simulink model "Complete_Sensorless_FOC_EKF_simulink_model"  (R2026a)
settings: Solver=ode23s  StopTime=inf  FixedStep=5e-5  MaxStep=1e-2
model workspace (MAT data in the model file):
  SL_ROS_VariableLengthArrays_MaxSizes : object (value not decoded)
values from neighbouring files (symbols this model uses):
  id_ref = 0    [motor_params.m]
  J = 0.001    [motor_params.m]
  Kp_id = 37.7    [motor_params.m]
  Kp_iq = 65.97    [motor_params.m]
  lam = 0.175    [motor_params.m]
  Ld = 6e-3    (= 0.006)    [motor_params.m]
  Lq = 10.5e-3    (= 0.0105)    [motor_params.m]
  Ts = 50e-6    (= 5e-05)    [motor_params.m]
  V_dc = 48    [motor_params.m]
  V_lim = 27.7    [motor_params.m]
undefined symbols (not defined in the file or in its folder): data, data_SL_Info, DiscIntNeverNeededParam, dspblkCoreblockFVToolHelper, gcbh
libraries: nesl_utility x34, fl_lib x22, ee_lib x16, ros2lib x3
(part 2 of 2)

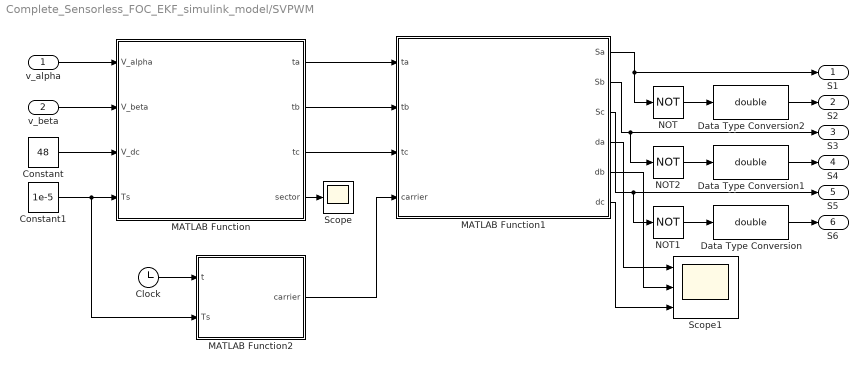
== system Complete_Sensorless_FOC_EKF_simulink_model/SVPWM ==
  v_alpha : Inport
  v_beta : Inport  Port=2
  Clock : Clock
  Constant : Constant  Value=48
  Constant1 : Constant  Value=1e-5
  Data Type Conversion : DataTypeConversion  OutDataTypeStr=double  SaturateOnIntegerOverflow=off  RndMeth=Floor
  Data Type Conversion1 : DataTypeConversion  OutDataTypeStr=double  SaturateOnIntegerOverflow=off  RndMeth=Floor
  Data Type Conversion2 : DataTypeConversion  OutDataTypeStr=double  SaturateOnIntegerOverflow=off  RndMeth=Floor
  MATLAB Function : MATLAB Function  TreatAsAtomicUnit=on
  MATLAB Function1 : MATLAB Function  TreatAsAtomicUnit=on
  MATLAB Function2 : MATLAB Function  TreatAsAtomicUnit=on
  NOT : Logic  Operator=NOT  IconShape=distinctive  AllPortsSameDT=off  OutDataTypeStr=boolean
  NOT1 : Logic  Operator=NOT  IconShape=distinctive  AllPortsSameDT=off  OutDataTypeStr=boolean
  NOT2 : Logic  Operator=NOT  IconShape=distinctive  AllPortsSameDT=off  OutDataTypeStr=boolean
  Scope : Scope
      settings: ActiveDisplayYMinimum=-1.4009794226019459  ActiveDisplayYMaximum=12.404458534659673
  Scope1 : Scope  NumInputPorts=3
      settings: ActiveDisplayYMinimum=-0.1185846672948957  ActiveDisplayYMaximum=0.92580647336062072  DataLoggingVariableName=ScopeData9
  S1 : Outport
  S2 : Outport  Port=2
  S3 : Outport  Port=3
  S4 : Outport  Port=4
  S5 : Outport  Port=5
  S6 : Outport  Port=6
  wires:
  v_alpha/1 -> MATLAB Function/1(V_alpha)
  v_beta/1 -> MATLAB Function/2(V_beta)
  Constant/1 -> MATLAB Function/3(V_dc)
  Constant1/1 -> MATLAB Function2/2(Ts), MATLAB Function/4(Ts)
  Clock/1 -> MATLAB Function2/1(t)
  MATLAB Function/1(ta) -> MATLAB Function1/1(ta)
  MATLAB Function/2(tb) -> MATLAB Function1/2(tb)
  MATLAB Function/3(tc) -> MATLAB Function1/3(tc)
  MATLAB Function2/1(carrier) -> MATLAB Function1/4(carrier)
  MATLAB Function1/2(Sb) -> NOT2/1, S3/1
  NOT/1 -> Data Type Conversion2/1
  NOT2/1 -> Data Type Conversion1/1
  NOT1/1 -> Data Type Conversion/1
  MATLAB Function/4(sector) -> Scope/1
  Data Type Conversion2/1 -> S2/1
  Data Type Conversion1/1 -> S4/1
  Data Type Conversion/1 -> S6/1
  MATLAB Function1/1(Sa) -> NOT/1, S1/1
  MATLAB Function1/3(Sc) -> NOT1/1, S5/1
  MATLAB Function1/4(da) -> Scope1/1
  MATLAB Function1/5(db) -> Scope1/2
  MATLAB Function1/6(dc) -> Scope1/3

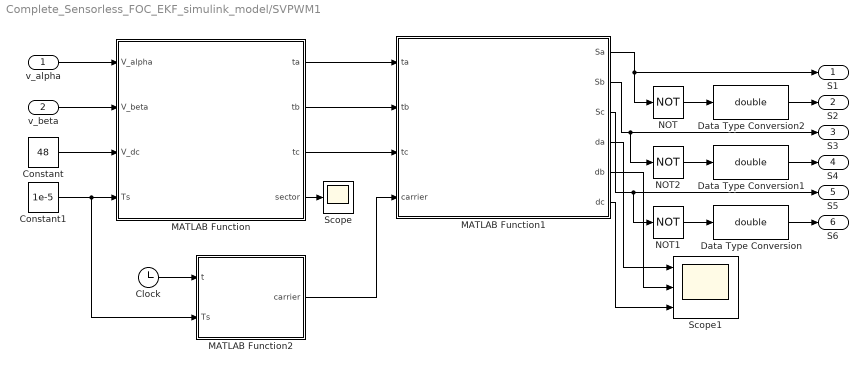
== system Complete_Sensorless_FOC_EKF_simulink_model/SVPWM1 ==
  v_alpha : Inport
  v_beta : Inport  Port=2
  Clock : Clock
  Constant : Constant  Value=48  SampleTime=-1
  Constant1 : Constant  Value=1e-5
  Data Type Conversion : DataTypeConversion  OutDataTypeStr=double  SaturateOnIntegerOverflow=off  RndMeth=Floor
  Data Type Conversion1 : DataTypeConversion  OutDataTypeStr=double  SaturateOnIntegerOverflow=off  RndMeth=Floor
  Data Type Conversion2 : DataTypeConversion  OutDataTypeStr=double  SaturateOnIntegerOverflow=off  RndMeth=Floor
  MATLAB Function : MATLAB Function  TreatAsAtomicUnit=on
  MATLAB Function1 : MATLAB Function  TreatAsAtomicUnit=on
  MATLAB Function2 : MATLAB Function  TreatAsAtomicUnit=on
  NOT : Logic  Operator=NOT  IconShape=distinctive  AllPortsSameDT=off  OutDataTypeStr=boolean
  NOT1 : Logic  Operator=NOT  IconShape=distinctive  AllPortsSameDT=off  OutDataTypeStr=boolean
  NOT2 : Logic  Operator=NOT  IconShape=distinctive  AllPortsSameDT=off  OutDataTypeStr=boolean
  Scope : Scope
      settings: ActiveDisplayYMinimum=-1.4009794226019459  ActiveDisplayYMaximum=12.404458534659673
  Scope1 : Scope  NumInputPorts=3
      settings: ActiveDisplayYMinimum=-0.1185846672948957  ActiveDisplayYMaximum=0.92580647336062072  DataLoggingVariableName=ScopeData9
  S1 : Outport
  S2 : Outport  Port=2
  S3 : Outport  Port=3
  S4 : Outport  Port=4
  S5 : Outport  Port=5
  S6 : Outport  Port=6
  wires:
  v_alpha/1 -> MATLAB Function/1(V_alpha)
  v_beta/1 -> MATLAB Function/2(V_beta)
  Constant/1 -> MATLAB Function/3(V_dc)
  Constant1/1 -> MATLAB Function2/2(Ts), MATLAB Function/4(Ts)
  Clock/1 -> MATLAB Function2/1(t)
  MATLAB Function/1(ta) -> MATLAB Function1/1(ta)
  MATLAB Function/2(tb) -> MATLAB Function1/2(tb)
  MATLAB Function/3(tc) -> MATLAB Function1/3(tc)
  MATLAB Function2/1(carrier) -> MATLAB Function1/4(carrier)
  MATLAB Function1/2(Sb) -> NOT2/1, S3/1
  NOT/1 -> Data Type Conversion2/1
  NOT2/1 -> Data Type Conversion1/1
  NOT1/1 -> Data Type Conversion/1
  MATLAB Function/4(sector) -> Scope/1
  Data Type Conversion2/1 -> S2/1
  Data Type Conversion1/1 -> S4/1
  Data Type Conversion/1 -> S6/1
  MATLAB Function1/1(Sa) -> NOT/1, S1/1
  MATLAB Function1/3(Sc) -> NOT1/1, S5/1
  MATLAB Function1/4(da) -> Scope1/1
  MATLAB Function1/5(db) -> Scope1/2
  MATLAB Function1/6(dc) -> Scope1/3

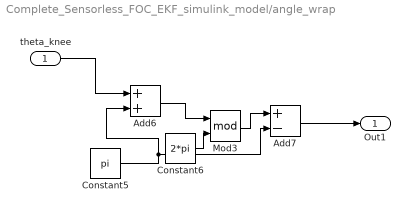
== system Complete_Sensorless_FOC_EKF_simulink_model/angle_wrap ==
  theta_knee : Inport
  Add6 : Sum
  Add7 : Sum  Inputs=+-
  Constant5 : Constant  Value=pi
  Constant6 : Constant  Value=2*pi
  Mod3 : Math  Operator=mod
  Out1 : Outport
  wires:
  Add6/1 -> Mod3/1
  Constant5/1 -> Add7/2, Add6/2
  Constant6/1 -> Mod3/2
  Mod3/1 -> Add7/1
  theta_knee/1 -> Add6/1
  Add7/1 -> Out1/1

== system Complete_Sensorless_FOC_EKF_simulink_model/angle_wrap1 ==
  theta_hip : Inport
  Add4 : Sum
  Add5 : Sum  Inputs=+-
  Constant : Constant  Value=pi
  Constant4 : Constant  Value=2*pi
  Mod2 : Math  Operator=mod
  Out1 : Outport
  wires:
  Add5/1 -> Out1/1
  Constant4/1 -> Mod2/2
  Constant/1 -> Add5/2, Add4/2
  Mod2/1 -> Add5/1
  theta_hip/1 -> Add4/1
  Add4/1 -> Mod2/1

== matlab function Complete_Sensorless_FOC_EKF_simulink_model/Inverse_park1 ==
  data: vd input; v_alpha output; vq input; theta input; v_beta output
function [v_alpha, v_beta] = inv_park_transform(vd, vq, theta)
v_alpha = vd * cos(theta) - vq * sin(theta);
v_beta  = vd * sin(theta) + vq * cos(theta);
end

== matlab function Complete_Sensorless_FOC_EKF_simulink_model/MATLAB Function2 ==
  settings: updateMethod=DISCRETE
  data: Ialpha_filt input; theta_hat output; Ibeta_filt input; Valpha input; Vbeta input; omega_hat output; Vdc input
function [theta_hat, omega_hat] = EKF_BackEMF(Ialpha_filt, Ibeta_filt, Valpha,Vbeta, Vdc)
%#codegen

% --- Motor & System Constants ---
Rs       = 2.875;
lambda_m = 0.175;
L_avg    = (6e-3 + 10.5e-3) / 2; % Ld/Lq average
dt       = 1e-5;

% Tuning Parameters
Q = diag([1e-6, 1e-3]);   % Process noise covariance
R = diag([1e-1, 1e-1]);   % Measurement noise covariance

% --- 1. Phase Voltage Reconstruction & Clarke Transform ---


% --- 2. Persistent State Initialization ---
persistent x P initialized
if isempty(initialized)
    x           = [0.0; 10.0];         % x = [theta_e; omega_e]
    P           = diag([1.0, 100.0]);
    initialized = true;
end

% --- 3. EKF Prediction Step ---
F      = [1.0, dt; 0.0, 1.0];
x_pred = F * x;
P_pred = F * P * F' + Q;

% Soft-clamp predicted electrical speed
omega_max_elec = 2*pi*1000; % Rad/s elec limit
x_pred(2) = max(min(x_pred(2), omega_max_elec), -omega_max_elec);

% Wrap predicted angle to [-pi, pi]
x_pred(1) = mod(x_pred(1) + pi, 2*pi) - pi;

% --- 4. Back-EMF Measurement Computation ---
% Measured Back-EMF from stator voltage equation (negligible L*di/dt)
e_alpha_meas = Valpha - Rs*Ialpha_filt;
e_beta_meas  = Vbeta  - Rs*Ibeta_filt;

% Modelled Back-EMF vector h(x)
theta_p = x_pred(1);
omega_p = x_pred(2);

h = [-omega_p * lambda_m * sin(theta_p);
      omega_p * lambda_m * cos(theta_p)];

% Measurement Jacobian H = dh/dx
H = [-omega_p * lambda_m * cos(theta_p), -lambda_m * sin(theta_p);
     -omega_p * lambda_m * sin(theta_p),  lambda_m * cos(theta_p)];

% --- 5. Measurement Update Step ---
y = [e_alpha_meas; e_beta_meas] - h;
S = H * P_pred * H' + R;

% Innovation Gate / Outlier Rejection
persistent y_reject_count
if isempty(y_reject_count)
    y_reject_count = 0;
end

d2 = y' * (S \ y);          
gate_threshold = 15;         
max_consecutive_rejects = 5; 

if d2 > gate_threshold && y_reject_count < max_consecutive_rejects
    x_new = x_pred;
    P_new = P_pred;
    y_reject_count = y_reject_count + 1;
else
    K     = (P_pred * H') / S;
    x_new = x_pred + K * y;
    
    IKH   = eye(2) - K * H;
    P_new = IKH * P_pred * IKH' + K * R * K';
    P_new = (P_new + P_new') / 2;
    y_reject_count = 0;
end

% --- 6. State Normalization & Output Assignment ---
% Wrap angle state to [-pi, pi]
x_new(1) = mod(x_new(1) + pi, 2*pi) - pi;

x = x_new;
P = P_new;

% Outputs (Electrical quantities directly suited for FOC Park/Clarke)
theta_hat = x(1); 
omega_hat = x(2); % NO -1 MULTIPLICATION

end

== matlab function Complete_Sensorless_FOC_EKF_simulink_model/MOTOR1/MATLAB Function ==
  data: id input; Te output; iq input
function Te = calc_torque(id, iq)
P   = 4;
lam = 0.175;
ld=6e-3;
lq=10.5e-3;
Te  = 1.5 * P * (lam*iq+(ld-lq)*id*iq);
end

== matlab function Complete_Sensorless_FOC_EKF_simulink_model/SVPWM1/MATLAB Function ==
  data: V_alpha input; ta output; V_beta input; V_dc input; Ts input; tb output; tc output; sector output
function [ta, tb, tc, sector] = fcn(V_alpha, V_beta, V_dc, Ts)
%#codegen

V_ref  = sqrt(V_alpha^2 + V_beta^2 + eps);
theta  = atan2(V_beta, V_alpha);
theta  = mod(theta, 2*pi);
if theta < 0; theta = theta + 2*pi; end

sector = floor(theta/(pi/3)) + 1;
if sector > 6; sector = 1; end

theta_s = theta - (sector-1)*(pi/3);
theta_s = max(0, min(pi/3, theta_s));

m  = min(sqrt(3)*V_ref/V_dc, 1.0);
T1 = Ts * m * sin(pi/3 - theta_s);
T2 = Ts * m * sin(theta_s);
T0 = Ts - T1 - T2;

if T0 < 0
    sc = Ts/(T1+T2);
    T1=T1*sc; T2=T2*sc; T0=0;
end

T0_4 = T0/4;
switch sector
    case 1; ta=T0_4;           tb=T0_4+T1/2;       tc=T0_4+T1/2+T2/2;
    case 2; ta=T0_4+T2/2;      tb=T0_4;            tc=T0_4+T1/2+T2/2;
    case 3; ta=T0_4+T1/2+T2/2; tb=T0_4;            tc=T0_4+T1/2;
    case 4; ta=T0_4+T1/2+T2/2; tb=T0_4+T2/2;       tc=T0_4;
    case 5; ta=T0_4+T1/2;      tb=T0_4+T1/2+T2/2;  tc=T0_4;
    case 6; ta=T0_4;           tb=T0_4+T1/2+T2/2;  tc=T0_4+T2/2;
    otherwise; ta=T0/2; tb=T0/2; tc=T0/2;
end
end

== matlab function Complete_Sensorless_FOC_EKF_simulink_model/SVPWM1/MATLAB Function1 ==
  data: ta input; Sa output; tb input; tc input; carrier input; Sb output; Sc output; da output; db output; dc output
function [Sa, Sb, Sc, da, db, dc] = fcn(ta, tb, tc, carrier)
Sa = double(carrier > ta);
Sb = double(carrier > tb);
Sc = double(carrier > tc);
Ts=1e-5;
da = ta / (Ts/2);   % Phase A duty cycle (0 to 1)
db = tb / (Ts/2);   % Phase B duty cycle
dc = tc / (Ts/2);   % Phase C duty cycle
end

== matlab function Complete_Sensorless_FOC_EKF_simulink_model/clarke ==
  data: ia input; i_alpha output; ib input; i_beta output
function [i_alpha, i_beta] = clarke_transform(ia, ib)
i_alpha = (2/3) * (ia - 0.5*ib - 0.5*(-(ia+ib)));
i_beta  = (2/3) * (sqrt(3)/2 * ib - sqrt(3)/2 * (-(ia+ib)));
end

== matlab function Complete_Sensorless_FOC_EKF_simulink_model/SVPWM1/MATLAB Function2 ==
  data: t input; carrier output; Ts input
function carrier = fcn(t, Ts)
%#codegen
phase   = mod(t, Ts) / Ts;
carrier = (Ts/2) * (1 - abs(2*phase - 1));
end

== matlab function Complete_Sensorless_FOC_EKF_simulink_model/clarke1 ==
  data: ia input; i_alpha output; ib input; i_beta output
function [i_alpha, i_beta] = clarke_transform(ia, ib)
i_alpha = (2/3) * (ia - 0.5*ib - 0.5*(-(ia+ib)));
i_beta  = (2/3) * (sqrt(3)/2 * ib - sqrt(3)/2 * (-(ia+ib)));
end

== matlab function Complete_Sensorless_FOC_EKF_simulink_model/park1 ==
  data: i_alpha input; id output; i_beta input; theta input; iq output
function [id, iq] = park_transform(i_alpha, i_beta, theta)
id =  i_alpha * cos(theta) + i_beta * sin(theta);
iq = -i_alpha * sin(theta) + i_beta * cos(theta);
end

== matlab function Complete_Sensorless_FOC_EKF_simulink_model/MOTOR/MATLAB Function ==
  data: id input; Te output; iq input
function Te = calc_torque(id, iq)
P   = 4;
lam = 0.175;
ld=6e-3;
lq=10.5e-3;
Te  = 1.5 * P * (lam*iq+(ld-lq)*id*iq);
end

== matlab function Complete_Sensorless_FOC_EKF_simulink_model/park ==
  data: i_alpha input; id output; i_beta input; theta input; iq output
function [id, iq] = park_transform(i_alpha, i_beta, theta)
id =  i_alpha * cos(theta) + i_beta * sin(theta);
iq = -i_alpha * sin(theta) + i_beta * cos(theta);
end

== matlab function Complete_Sensorless_FOC_EKF_simulink_model/Inverse_park ==
  data: vd input; v_alpha output; vq input; theta input; v_beta output
function [v_alpha, v_beta] = inv_park_transform(vd, vq, theta)
v_alpha = vd * cos(theta) - vq * sin(theta);
v_beta  = vd * sin(theta) + vq * cos(theta);
end

== matlab function Complete_Sensorless_FOC_EKF_simulink_model/SVPWM/MATLAB Function ==
  data: V_alpha input; ta output; V_beta input; V_dc input; Ts input; tb output; tc output; sector output
function [ta, tb, tc, sector] = fcn(V_alpha, V_beta, V_dc, Ts)

V_ref  = sqrt(V_alpha^2 + V_beta^2 + eps);
theta  = atan2(V_beta, V_alpha);
theta  = mod(theta, 2*pi);
if theta < 0; theta = theta + 2*pi; end

sector = floor(theta/(pi/3)) + 1;
if sector > 6; sector = 1; end

theta_s = theta - (sector-1)*(pi/3);
theta_s = max(0, min(pi/3, theta_s));

m  = min(sqrt(3)*V_ref/V_dc, 1.0);
T1 = Ts * m * sin(pi/3 - theta_s);
T2 = Ts * m * sin(theta_s);
T0 = Ts - T1 - T2;

if T0 < 0
    sc = Ts/(T1+T2);
    T1=T1*sc; T2=T2*sc; T0=0;
end

T0_4 = T0/4;
switch sector
    case 1; ta=T0_4;           tb=T0_4+T1/2;       tc=T0_4+T1/2+T2/2;
    case 2; ta=T0_4+T2/2;      tb=T0_4;            tc=T0_4+T1/2+T2/2;
    case 3; ta=T0_4+T1/2+T2/2; tb=T0_4;            tc=T0_4+T1/2;
    case 4; ta=T0_4+T1/2+T2/2; tb=T0_4+T2/2;       tc=T0_4;
    case 5; ta=T0_4+T1/2;      tb=T0_4+T1/2+T2/2;  tc=T0_4;
    case 6; ta=T0_4;           tb=T0_4+T1/2+T2/2;  tc=T0_4+T2/2;
    otherwise; ta=T0/2; tb=T0/2; tc=T0/2;
end
end

== matlab function Complete_Sensorless_FOC_EKF_simulink_model/SVPWM/MATLAB Function1 ==
  data: ta input; Sa output; tb input; tc input; carrier input; Sb output; Sc output; da output; db output; dc output
function [Sa, Sb, Sc, da, db, dc] = fcn(ta, tb, tc, carrier)
Sa = double(carrier > ta);
Sb = double(carrier > tb);
Sc = double(carrier > tc);
Ts=1e-5;
da = ta / (Ts/2);   % Phase A duty cycle (0 to 1)
db = tb / (Ts/2);   % Phase B duty cycle
dc = tc / (Ts/2);   % Phase C duty cycle
end

== matlab function Complete_Sensorless_FOC_EKF_simulink_model/SVPWM/MATLAB Function2 ==
  data: t input; carrier output; Ts input
function carrier = fcn(t, Ts)
phase   = mod(t, Ts) / Ts;
carrier = (Ts/2) * (1 - abs(2*phase - 1));
end

== matlab function Complete_Sensorless_FOC_EKF_simulink_model/MATLAB Function1 ==
  settings: updateMethod=DISCRETE
  data: Ialpha_filt input; theta_hat output; Ibeta_filt input; Valpha input; Vbeta input; omega_hat output; Vdc input
function [theta_hat, omega_hat] = EKF_BackEMF(Ialpha_filt, Ibeta_filt, Valpha,Vbeta, Vdc)
%#codegen

% --- Motor & System Constants ---
Rs       = 2.875;
lambda_m = 0.175;
L_avg    = (6e-3 + 10.5e-3) / 2; % Ld/Lq average
dt       = 1e-5;

% Tuning Parameters
Q = diag([1e-6, 1e-3]);   % Process noise covariance
R = diag([1e-1, 1e-1]);   % Measurement noise covariance

% --- 1. Phase Voltage Reconstruction & Clarke Transform ---


% --- 2. Persistent State Initialization ---
persistent x P initialized
if isempty(initialized)
    x           = [0.0; 10.0];         % x = [theta_e; omega_e]
    P           = diag([1.0, 100.0]);
    initialized = true;
end

% --- 3. EKF Prediction Step ---
F      = [1.0, dt; 0.0, 1.0];
x_pred = F * x;
P_pred = F * P * F' + Q;

% Soft-clamp predicted electrical speed
omega_max_elec = 2*pi*1000; % Rad/s elec limit
x_pred(2) = max(min(x_pred(2), omega_max_elec), -omega_max_elec);

% Wrap predicted angle to [-pi, pi]
x_pred(1) = mod(x_pred(1) + pi, 2*pi) - pi;

% --- 4. Back-EMF Measurement Computation ---
% Measured Back-EMF from stator voltage equation (negligible L*di/dt)
e_alpha_meas = Valpha - Rs*Ialpha_filt;
e_beta_meas  = Vbeta  - Rs*Ibeta_filt;

% Modelled Back-EMF vector h(x)
theta_p = x_pred(1);
omega_p = x_pred(2);

h = [-omega_p * lambda_m * sin(theta_p);
      omega_p * lambda_m * cos(theta_p)];

% Measurement Jacobian H = dh/dx
H = [-omega_p * lambda_m * cos(theta_p), -lambda_m * sin(theta_p);
     -omega_p * lambda_m * sin(theta_p),  lambda_m * cos(theta_p)];

% --- 5. Measurement Update Step ---
y = [e_alpha_meas; e_beta_meas] - h;
S = H * P_pred * H' + R;

% Innovation Gate / Outlier Rejection
persistent y_reject_count
if isempty(y_reject_count)
    y_reject_count = 0;
end

d2 = y' * (S \ y);          
gate_threshold = 15;         
max_consecutive_rejects = 5; 

if d2 > gate_threshold && y_reject_count < max_consecutive_rejects
    x_new = x_pred;
    P_new = P_pred;
    y_reject_count = y_reject_count + 1;
else
    K     = (P_pred * H') / S;
    x_new = x_pred + K * y;
    
    IKH   = eye(2) - K * H;
    P_new = IKH * P_pred * IKH' + K * R * K';
    P_new = (P_new + P_new') / 2;
    y_reject_count = 0;
end

% --- 6. State Normalization & Output Assignment ---
% Wrap angle state to [-pi, pi]
x_new(1) = mod(x_new(1) + pi, 2*pi) - pi;

x = x_new;
P = P_new;

% Outputs (Electrical quantities directly suited for FOC Park/Clarke)
theta_hat = x(1); 
omega_hat = x(2); % NO -1 MULTIPLICATION

end
